simulink model "ADCOut"  (R2017a)
settings: Solver=VariableStepAuto  StartTime=0.0  StopTime=10.0  RelTol=1e-3
values from neighbouring files (symbols this model uses):
  gainCapteur = 12./max(abs(SortieCapteur(:,2)))    [problematiqueM.m]
libraries: dsparch4 x1, simulink_extras x1
settings Model: Creator=Guacamole  LastModifiedBy=Guacamole

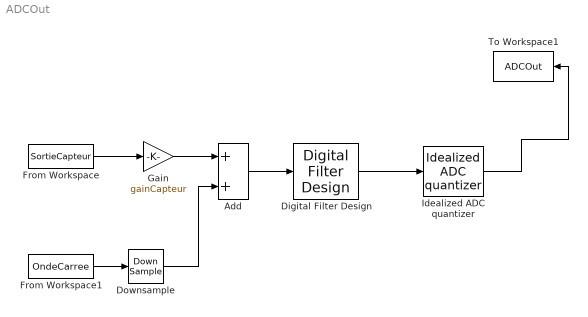
== system ADCOut ==
  Add : Sum
  Digital Filter Design : dsparch4/Digital Filter Design  mwdsp_browser_bugfix_var=off
  Downsample : DownSample  N=3  RateOptions=Allow multirate processing
  From Workspace : FromWorkspace  VariableName=SortieCapteur  SampleTime=1/16000  Interpolate=off  OutputAfterFinalValue=Setting to zero
  From Workspace1 : FromWorkspace  VariableName=OndeCarree  SampleTime=1/48000  Interpolate=off  OutputAfterFinalValue=Setting to zero
  Gain : Gain  Gain=gainCapteur
  Idealized ADC quantizer : simulink_extras/Additional Discrete/Idealized ADC quantizer  NumberOfConverterBits=10  Vmin=-12  Vmax=12  OutputDataType=double  OutputNegativeValues=on
      settings: SourceProductName=Simulink
  To Workspace1 : ToWorkspace  VariableName=ADCOut  SampleTime=-1
      settings: Save2DSignal=2-D array (concatenate along first dimension)
  wires:
  From Workspace/1 -> Gain/1
  Gain/1 -> Add/1
  Digital Filter Design/1 -> Idealized ADC quantizer/1
  From Workspace1/1 -> Downsample/1
  Add/1 -> Digital Filter Design/1
  Idealized ADC quantizer/1 -> To Workspace1/1
  Downsample/1 -> Add/2
